simulink model "Practica2_1"  (R2018b)
settings: Solver=VariableStepAuto  StartTime=0.0  StopTime=100  RelTol=1e-3
settings Model: Creator=ramon  LastModifiedBy=ramon

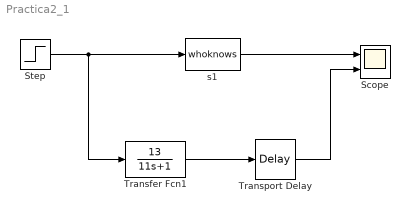
== system Practica2_1 ==
  Scope : Scope  NumInputPorts=2
  Step : Step  SampleTime=0
  Transfer Fcn1 : TransferFcn  Numerator=13  Denominator=[11 1]
  Transport Delay : TransportDelay
  s1 : M-S-Function  FunctionName=whoknows  Parameters=L, P1, P2, T, R  mask{L=7, P1=0, P2=9, T=1, R=0}
      mask prompts: L "Laboratorio"; P1 "Primer digito del Puesto"; P2 "Segundo digito del Puesto"; T "Tipo de Planta"; R "Ruido"
      mask Display: disp('Sistema')
  wires:
  s1/1 -> Scope/1
  Transport Delay/1 -> Scope/2
  Step/1 -> Transfer Fcn1/1, s1/1
  Transfer Fcn1/1 -> Transport Delay/1
